simulink model "Problem_5"  (R2020a)
settings: Solver=VariableStepAuto  StartTime=0.0  StopTime=10  RelTol=1e-3
model workspace (MAT data in the model file):
  C = 1e-06
  E = 100
  R = 10
settings Model: Creator=Shubham Singh Rathor  LastModifiedBy=Shubham Singh Rathor

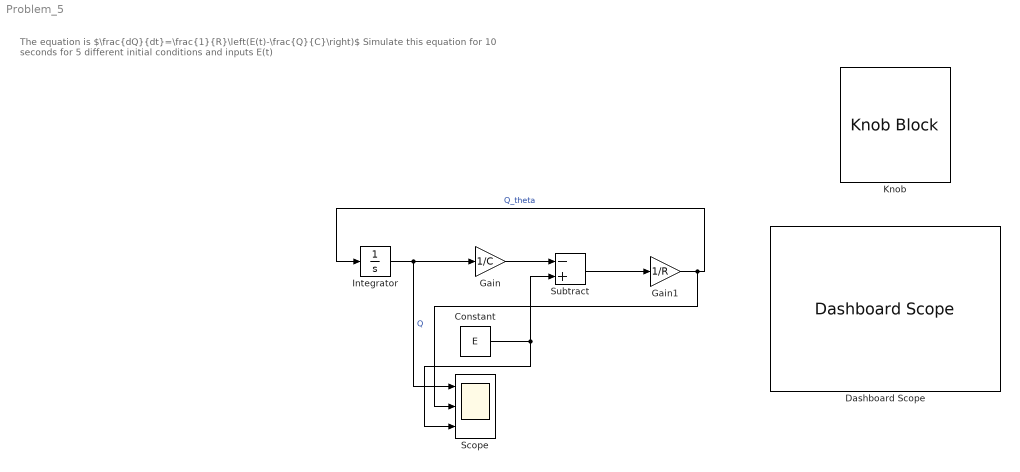
== system Problem_5 ==
  note: The equation is
      | $\frac{dQ}{dt}=\frac{1}{R}\left(E(t)-\frac{Q}{C}\right)$
      | Simulate this equation for 10 seconds for 5 different initial conditions and inputs E(t)
  Constant : Constant  Value=E
  Dashboard Scope : DashboardScope
  Gain : Gain  Gain=1/C
  Gain1 : Gain  Gain=1/R
  Integrator : Integrator
  Knob : KnobBlock
  Scope : Scope  NumInputPorts=3
  Subtract : Sum  Inputs=-+
  wires:
  Integrator/1 -> Scope/1, Gain/1  "Q"
  Gain1/1 -> Scope/2, Integrator/1  "Q_theta"
  Gain/1 -> Subtract/1
  Constant/1 -> Scope/3, Subtract/2
  Subtract/1 -> Gain1/1
